simulink model "B_sim_matrix"  (R2016b)
settings: Solver=ode45  StartTime=0.0  StopTime=10.0  RelTol=1e-3  EnableMultiTasking=on
values from neighbouring files (symbols this model uses):
  a_1 = 1    [parameters.m]
  I_l_1 = 10    [parameters.m]
  I_l_2 = 10    [parameters.m]
  I_m_1 = 0.01    [parameters.m]
  I_m_2 = 0.01    [parameters.m]
  k_r_1 = 100    [parameters.m]
  k_r_2 = 100    [parameters.m]
  l_1 = 0.5    [parameters.m]
  l_2 = 0.5    [parameters.m]
  m_l_1 = 50    [parameters.m]
  m_l_2 = 50    [parameters.m]
  m_m_2 = 5    [parameters.m]
settings Model: Creator=kma  LastModifiedBy=kma
settings DataIOCC: LimitDataPoints=on  SaveFormat=Array
settings OptimizationCC: LifeSpan=inf
settings DebuggingCC: SFUnexpectedBacktrackingDiag=warning  SFNoUnconditionalDefaultTransitionDiag=warning  SFExecutionAtInitializationDiag=none
settings HardwareCC: ProdBitPerPointer=32  ProdBitPerSizeT=32  ProdBitPerPtrDiffT=32  ProdLargestAtomicFloat=None  ProdIntDivRoundTo=Undefined  ProdEndianess=Unspecified  ProdWordSize=32  ProdHWDeviceType=32-bit Generic
settings ModelReferenceCC: PropagateSignalLabelsOutOfModel=off
settings GRTTargetCC: TargetLangStandard=C89/C90 (ANSI)  GeneratePreprocessorConditionals=Disable all
settings ConfigComp: CovMetricSettings=dw  CovHtmlReporting=on  CovSaveCumulativeToWorkspaceVar=on  CovSaveSingleToWorkspaceVar=on  CovExternalEMLEnable=off

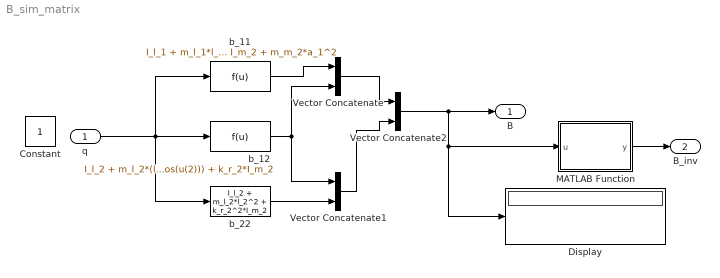
== system B_sim_matrix ==
  q : Inport  PortDimensions=2
  Display : Display
  MATLAB Function : MATLAB Function  TreatAsAtomicUnit=on
  Vector Concatenate : Concatenate
  Vector Concatenate1 : Concatenate
  Vector Concatenate2 : Concatenate  Mode=Multidimensional array  ConcatenateDimension=2
  b_11 : Fcn  Expr=I_l_1 + m_l_1*l_1^2 + k_r_1^2*I_m_1 + I_l_2 + m_l_2*(a_1^2 + l_2^2 + 2*a_1*l_2*cos(u(2))) + I_m_2 + m_m_2*a_1^2
  b_12 : Fcn  Expr=I_l_2 + m_l_2*(l_2^2 + a_1*l_2*cos(u(2))) + k_r_2*I_m_2
  b_22 : Fcn  Expr=I_l_2 + m_l_2*l_2^2 + k_r_2^2*I_m_2
  B : Outport
  B_inv : Outport  Port=2
  Constant : Constant  IOType=siggen
  wires:
  q/1 -> b_22/1, b_12/1, b_11/1
  b_11/1 -> Vector Concatenate/1
  b_12/1 -> Vector Concatenate1/1, Vector Concatenate/2
  b_22/1 -> Vector Concatenate1/2
  Vector Concatenate/1 -> Vector Concatenate2/1
  Vector Concatenate1/1 -> Vector Concatenate2/2
  Vector Concatenate2/1 -> MATLAB Function/1(u), Display/1, B/1
  MATLAB Function/1(y) -> B_inv/1

== matlab function B_sim_matrix/MATLAB Function ==
  data: u input; y output
function y = fcn(u)
%#codegen

y = inv(u);
